simulink library "hEemethod"  (R2017b)
settings: Solver=VariableStepAuto  StartTime=0.0  StopTime=10.0  RelTol=1e-3
undefined symbols (not defined in the file or in its folder): Mag, r0_follower, v0_follower
libraries: hEemethod x13, vrlib x4, sharedutil x1, simulink x1
settings Model: Creator=mtwal  LastModifiedBy=mtwal
settings CodeAppCC: StateflowObjectComments=on

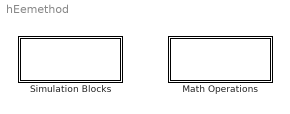
== system hEemethod ==
  Math Operations : Subsystem
  Simulation Blocks : Subsystem

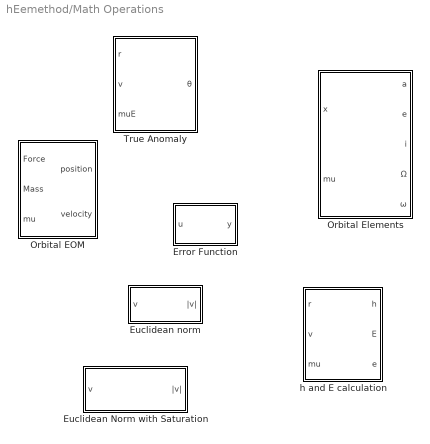
== system hEemethod/Math Operations ==
  Error Function : Subsystem  mask(Error Function){}
      mask help: Computes the error function of input signal u.
  Euclidean Norm with Saturation : Subsystem  mask(Euclidean Norm with Saturation){}
      mask help: Euclidean norm with minimum value of 1e-10 to avoid noise amplification at small values and maximum value of 1e20 to avoid infinity errors
  Euclidean norm : Subsystem  mask(Euclidean Norm){}
      mask help: Gives the Euclidean norm of a vector input
  Orbital EOM : Subsystem  mask(Orbit EOM){}
      mask help: Computes orbital EOM
  Orbital Elements : Subsystem  mask(Orbital Elements){}
      mask help: Calculates orbital elements from state vector x and gravitational constant mu
  True Anomaly : Subsystem  mask(True Anomaly){}
      mask help: Calculates true anomaly for given position, velocity, and planetary body
  h and E calculation : Subsystem  mask(hEe Calculation){}
      mask help: Calculate angular momentum (h), orbital energy (E), and eccentricity (e) for given postion, velocity, and gravitational constant

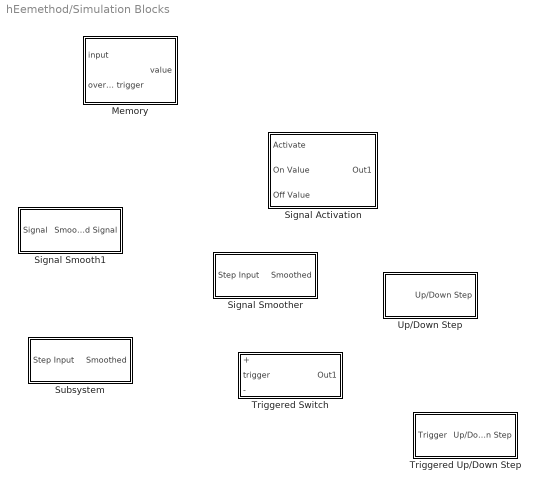
== system hEemethod/Simulation Blocks ==
  Memory : Subsystem  mask(Memory){}
      mask help: Holds value of input signal when a the value of overwrite trigger signal becomes greater than 0
  Signal Activation : Subsystem  mask(Signal Activation){RampTime=1}
      mask prompts: RampTime "Time for signal to ramp from 0 to 1"
      mask help: Outputs a signal that smoothly ramps from the off value to the on value when the activation input becomes greater than zero, and then smoothly ramps from the on value to the off value when the activation input becomes less than zero.
  Signal Smooth1 : Subsystem
  Signal Smoother : Subsystem  mask(Signal Smoother){Mag=0}
      mask prompts: Mag "Magnitude of Output Signal"
      mask help: Smooth a step function using an Error Function as a smooth approximation
  Subsystem : Subsystem
  Triggered Switch : Subsystem  mask(Triggered Switch){}
      mask help: Switches between + and - signal upon a triggering event
  Triggered Up/Down Step : Subsystem  mask(Triggered Up/Down Step){}
      mask help: Step up on rising trigger event and step down on falling trigger event
  Up/Down Step : Subsystem  mask(Up/Down Step){Mag1=0, tstep1=0, Mag2=0, tstep2=0}
      mask prompts: Mag1 "Magnitude of Positive Step Function"; tstep1 "Step Time of Positive Step Function"; Mag2 "Magnitude of Negative Step Function"; tstep2 "Step Time of Negative Step Function"
      mask help: Outputs a positive then a negative step function with specified magnitudes and step times.
      mask DialogControl Mag1 Tooltip: Magnitude of Positive Step
      mask DialogControl tstep1 Tooltip: Time of Positive Step
      mask DialogControl Mag2 Tooltip: Magnitude of Negative Step
      mask DialogControl tstep2 Tooltip: Step Time of Negative Step

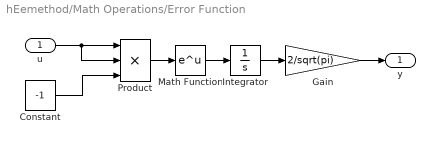
== system hEemethod/Math Operations/Error Function ==
  u : Inport
  Constant : Constant  Value=-1
  Gain : Gain  Gain=2/sqrt(pi)
  Integrator : Integrator
  Math Function : Math  SaturateOnIntegerOverflow=on
  Product : Product  Inputs=3
  y : Outport
  wires:
  u/1 -> Product/2, Product/1
  Constant/1 -> Product/3
  Product/1 -> Math Function/1
  Math Function/1 -> Integrator/1
  Integrator/1 -> Gain/1
  Gain/1 -> y/1

== system hEemethod/Math Operations/Euclidean Norm with Saturation ==
  v : Inport
  Dot Product : DotProduct  InputSameDT=on  OutDataTypeStr=Inherit: Inherit via internal rule
  Math Function : Math  Operator=sqrt  SaturateOnIntegerOverflow=on
  Saturation : Saturate  UpperLimit=1e20  LowerLimit=1e-10
  |v| : Outport
  wires:
  Saturation/1 -> |v|/1
  Math Function/1 -> Saturation/1
  v/1 -> Dot Product/1, Dot Product/2
  Dot Product/1 -> Math Function/1

== system hEemethod/Math Operations/Euclidean norm ==
  v : Inport
  Dot Product : DotProduct  InputSameDT=on  OutDataTypeStr=Inherit: Inherit via internal rule
  Math Function : Math  Operator=sqrt  SaturateOnIntegerOverflow=on
  |v| : Outport
  wires:
  v/1 -> Dot Product/1, Dot Product/2
  Dot Product/1 -> Math Function/1
  Math Function/1 -> |v|/1

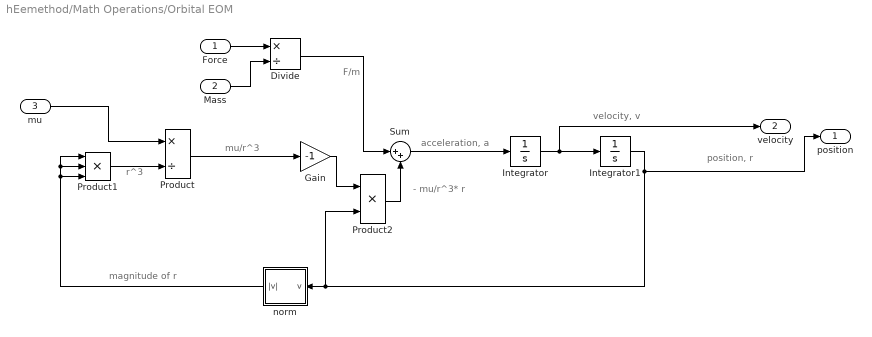
== system hEemethod/Math Operations/Orbital EOM ==
  note: F/m
  note: - mu/r^3* r
  note: mu/r^3
  note: r^3
  note: magnitude of r
  note: acceleration, a
  note: position, r
  note: velocity, v
  Force : Inport
  Mass : Inport  Port=2
  mu : Inport  Port=3
  Divide : Product  Inputs=*/
  Gain : Gain  Gain=-1  SaturateOnIntegerOverflow=on  OutDataTypeStr=Inherit: Same as input  ParamDataTypeStr=Inherit: Same as input
  Integrator : Integrator  InitialCondition=v0_follower  AbsoluteTolerance=1e-6
  Integrator1 : Integrator  InitialCondition=r0_follower  AbsoluteTolerance=1e-6
  Product : Product  Inputs=*/  SaturateOnIntegerOverflow=on  OutDataTypeStr=Inherit: Same as first input
  Product1 : Product  Inputs=***  SaturateOnIntegerOverflow=on  OutDataTypeStr=Inherit: Same as first input
  Product2 : Product  Inputs=**  SaturateOnIntegerOverflow=on  OutDataTypeStr=Inherit: Same as first input
  Sum : Sum  Inputs=|++
  norm : Subsystem
  position : Outport
  velocity : Outport  Port=2
  wires:
  mu/1 -> Product/1
  Product1/1 -> Product/2
  Integrator1/1 -> Product2/2, norm/1(v), position/1
  Product/1 -> Gain/1
  Integrator/1 -> Integrator1/1, velocity/1
  norm/1(|v|) -> Product1/1, Product1/2, Product1/3
  Gain/1 -> Product2/1
  Force/1 -> Divide/1
  Divide/1 -> Sum/1
  Product2/1 -> Sum/2
  Sum/1 -> Integrator/1
  Mass/1 -> Divide/2

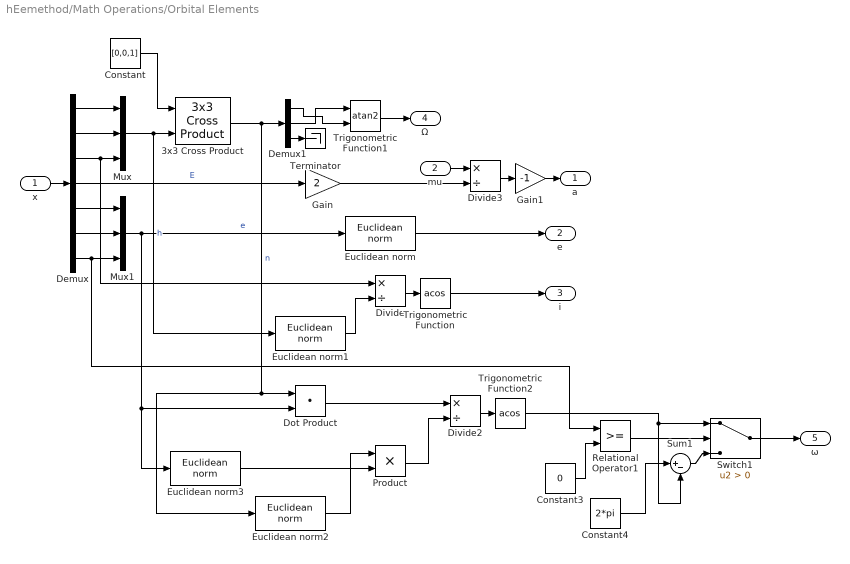
== system hEemethod/Math Operations/Orbital Elements ==
  x : Inport
  mu : Inport  Port=2
  3x3 Cross Product : sharedutil/3x3 Cross Product
      settings: SourceProductBaseCode=AE
  Constant : Constant  Value=[0,0,1]
  Constant3 : Constant  Value=0
  Constant4 : Constant  Value=2*pi
  Demux : Demux  Outputs=7
  Demux1 : Demux  Outputs=3
  Divide : Product  Inputs=*/
  Divide2 : Product  Inputs=*/
  Divide3 : Product  Inputs=*/
  Dot Product : DotProduct  InputSameDT=on  OutDataTypeStr=Inherit: Inherit via internal rule
  Euclidean norm{,1..3} (4 alike) : hEemethod/Math Operations/Euclidean norm
      settings: SourceProductName=HEe Method Library
  Gain : Gain  Gain=2
  Gain1 : Gain  Gain=-1
  Mux : Mux  Inputs=3
  Mux1 : Mux  Inputs=3
  Product : Product
  Relational Operator1 : RelationalOperator  OutDataTypeStr=boolean  RndMeth=Simplest
  Sum1 : Sum  Inputs=|+-
  Switch1 : Switch  Criteria=u2 > Threshold
  Terminator : Terminator
  Trigonometric Function : Trigonometry  Operator=acos
  Trigonometric Function1 : Trigonometry  Operator=atan2
  Trigonometric Function2 : Trigonometry  Operator=acos
  a : Outport
  e : Outport  Port=2
  i : Outport  Port=3
  Ω : Outport  Port=4
  ω : Outport  Port=5
  wires:
  Demux/1 -> Mux/1
  Demux/2 -> Mux/2
  Demux/3 -> Divide/1, Mux/3
  Demux/5 -> Mux1/1
  Demux/6 -> Mux1/2
  Demux/7 -> Relational Operator1/1, Mux1/3
  Demux/4 -> Gain/1  "E"
  Gain/1 -> Divide3/2
  Mux1/1 -> Euclidean norm/1, Euclidean norm3/1, Dot Product/2  "e"
  Euclidean norm/1 -> e/1
  Mux/1 -> Euclidean norm1/1, 3x3 Cross Product/2  "h"
  Constant/1 -> 3x3 Cross Product/1
  Divide/1 -> Trigonometric Function/1
  Euclidean norm1/1 -> Divide/2
  Trigonometric Function/1 -> i/1
  3x3 Cross Product/1 -> Demux1/1, Euclidean norm2/1, Dot Product/1  "n"
  Trigonometric Function1/1 -> Ω/1
  Euclidean norm3/1 -> Product/2
  Divide2/1 -> Trigonometric Function2/1
  Dot Product/1 -> Divide2/1
  Product/1 -> Divide2/2
  Sum1/1 -> Switch1/3
  Constant3/1 -> Relational Operator1/2
  Constant4/1 -> Sum1/1
  Relational Operator1/1 -> Switch1/2
  Switch1/1 -> ω/1
  Trigonometric Function2/1 -> Sum1/2, Switch1/1
  x/1 -> Demux/1
  mu/1 -> Divide3/1
  Gain1/1 -> a/1
  Divide3/1 -> Gain1/1
  Demux1/3 -> Terminator/1
  Demux1/2 -> Trigonometric Function1/1
  Demux1/1 -> Trigonometric Function1/2
  Euclidean norm2/1 -> Product/1

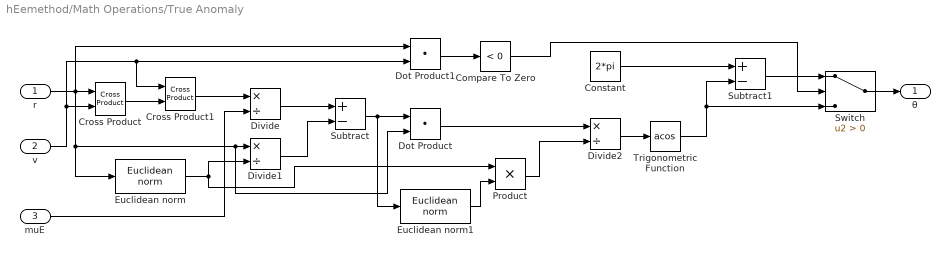
== system hEemethod/Math Operations/True Anomaly ==
  r : Inport
  v : Inport  Port=2
  muE : Inport  Port=3
  Compare To Zero : simulink/Logic and Bit Operations/Compare To Zero  relop=<  OutDataTypeStr=boolean
  Constant : Constant  Value=2*pi
  Cross Product : vrlib/Utilities/Cross Product
      settings: SourceProductBaseCode=VR
  Cross Product1 : vrlib/Utilities/Cross Product
      settings: SourceProductBaseCode=VR
  Divide : Product  Inputs=*/
  Divide1 : Product  Inputs=*/
  Divide2 : Product  Inputs=*/
  Dot Product : DotProduct  InputSameDT=on  OutDataTypeStr=Inherit: Inherit via internal rule
  Dot Product1 : DotProduct  InputSameDT=on  OutDataTypeStr=Inherit: Inherit via internal rule
  Euclidean norm : hEemethod/Math Operations/Euclidean norm
      settings: SourceProductName=HEe Method Library
  Euclidean norm1 : hEemethod/Math Operations/Euclidean norm
      settings: SourceProductName=HEe Method Library
  Product : Product
  Subtract : Sum  Inputs=+-
  Subtract1 : Sum  Inputs=+-
  Switch : Switch  Criteria=u2 > Threshold
  Trigonometric Function : Trigonometry  Operator=acos  OutputSignalType=real
  θ : Outport
  wires:
  r/1 -> Dot Product1/1, Dot Product/2, Divide1/1, Euclidean norm/1, Cross Product/1
  v/1 -> Cross Product/2, Cross Product1/1, Dot Product1/2
  Cross Product/1 -> Cross Product1/2
  Cross Product1/1 -> Divide/1
  muE/1 -> Divide/2
  Divide/1 -> Subtract/1
  Divide1/1 -> Subtract/2
  Euclidean norm/1 -> Product/1, Divide1/2
  Subtract/1 -> Euclidean norm1/1, Dot Product/1
  Dot Product/1 -> Divide2/1
  Product/1 -> Divide2/2
  Euclidean norm1/1 -> Product/2
  Dot Product1/1 -> Compare To Zero/1
  Constant/1 -> Subtract1/1
  Subtract1/1 -> Switch/1
  Compare To Zero/1 -> Switch/2
  Switch/1 -> θ/1
  Divide2/1 -> Trigonometric Function/1
  Trigonometric Function/1 -> Switch/3, Subtract1/2

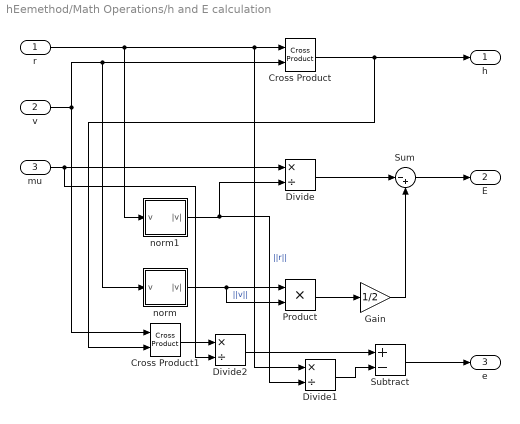
== system hEemethod/Math Operations/h and E calculation ==
  r : Inport
  v : Inport  Port=2
  mu : Inport  Port=3
  Cross Product : vrlib/Utilities/Cross Product
      settings: SourceProductBaseCode=VR
  Cross Product1 : vrlib/Utilities/Cross Product
      settings: SourceProductBaseCode=VR
  Divide : Product  Inputs=*/
  Divide1 : Product  Inputs=*/
  Divide2 : Product  Inputs=*/
  Gain : Gain  Gain=1/2
  Product : Product
  Subtract : Sum  Inputs=+-
  Sum : Sum  Inputs=|-+
  norm : Subsystem
  norm1 : Subsystem
  h : Outport
  E : Outport  Port=2
  e : Outport  Port=3
  wires:
  r/1 -> Divide1/1, Cross Product/1, norm1/1(v)
  v/1 -> Cross Product1/1, norm/1(v), Cross Product/2
  Cross Product/1 -> Cross Product1/2, h/1
  norm1/1(|v|) -> Divide1/2, Divide/2  "||r||"
  norm/1(|v|) -> Product/2, Product/1  "||v||"
  Product/1 -> Gain/1
  mu/1 -> Divide2/2, Divide/1
  Divide/1 -> Sum/1
  Gain/1 -> Sum/2
  Sum/1 -> E/1
  Divide1/1 -> Subtract/2
  Subtract/1 -> e/1
  Cross Product1/1 -> Divide2/1
  Divide2/1 -> Subtract/1

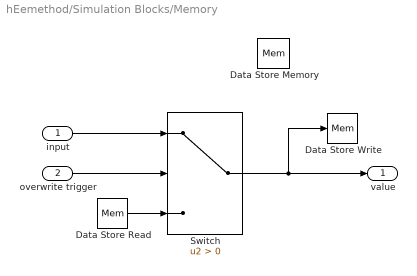
== system hEemethod/Simulation Blocks/Memory ==
  input : Inport
  overwrite trigger : Inport  Port=2
  Data Store Memory : DataStoreMemory  DataStoreName=Mem  ShowAdditionalParam=off
  Data Store Read : DataStoreRead  DataStoreName=Mem  SampleTime=[0,0]  DataStoreElements=Mem
  Data Store Write : DataStoreWrite  DataStoreName=Mem  SampleTime=[0,0]  DataStoreElements=Mem
  Switch : Switch  Criteria=u2 > Threshold
  value : Outport
  wires:
  Switch/1 -> Data Store Write/1, value/1
  input/1 -> Switch/1
  overwrite trigger/1 -> Switch/2
  Data Store Read/1 -> Switch/3

== system hEemethod/Simulation Blocks/Signal Activation ==
  Activate : Inport
  On Value : Inport  Port=2
  Off Value : Inport  Port=3
  Clock : Clock
  Memory : hEemethod/Simulation Blocks/Memory
      settings: SourceProductName=HEe Method Library
  Switch : Switch  Criteria=u2 > Threshold
  Out1 : Outport
  wires:
  Clock/1 -> ?
  Activate/1 -> Memory/2, Switch/2
  On Value/1 -> Switch/1
  Off Value/1 -> Switch/3
  Switch/1 -> Memory/1

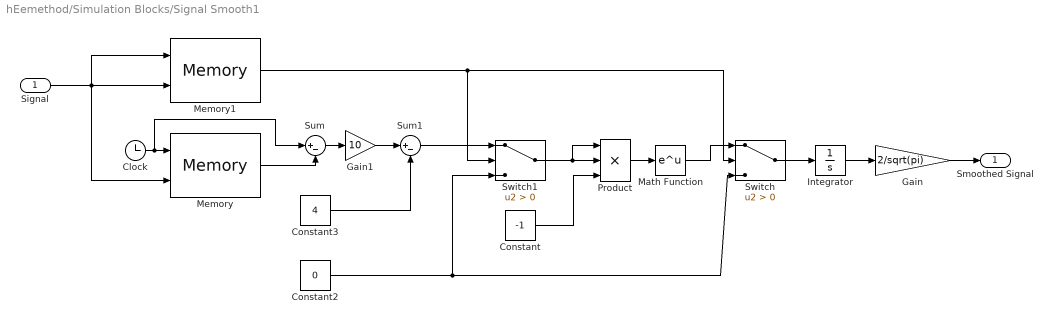
== system hEemethod/Simulation Blocks/Signal Smooth1 ==
  Signal : Inport
  Clock : Clock
  Constant : Constant  Value=-1
  Constant2 : Constant  Value=0
  Constant3 : Constant  Value=4
  Gain : Gain  Gain=2/sqrt(pi)
  Gain1 : Gain  Gain=10
  Integrator : Integrator
  Math Function : Math  SaturateOnIntegerOverflow=on
  Memory : hEemethod/Simulation Blocks/Memory
      settings: SourceProductName=HEe Method Library
  Memory1 : hEemethod/Simulation Blocks/Memory
      settings: SourceProductName=HEe Method Library
  Product : Product  Inputs=3
  Sum : Sum  Inputs=|+-
  Sum1 : Sum  Inputs=|+-
  Switch : Switch  Criteria=u2 > Threshold
  Switch1 : Switch  Criteria=u2 > Threshold
  Smoothed Signal : Outport
  wires:
  Memory/1 -> Sum/2
  Signal/1 -> Memory1/2, Memory1/1, Memory/2
  Clock/1 -> Sum/1, Memory/1
  Switch1/1 -> Product/1, Product/2
  Constant/1 -> Product/3
  Gain/1 -> Smoothed Signal/1
  Product/1 -> Math Function/1
  Integrator/1 -> Gain/1
  Switch/1 -> Integrator/1
  Math Function/1 -> Switch/1
  Memory1/1 -> Switch1/2, Switch/2
  Sum/1 -> Gain1/1
  Gain1/1 -> Sum1/1
  Sum1/1 -> Switch1/1
  Constant3/1 -> Sum1/2
  Constant2/1 -> Switch/3, Switch1/3

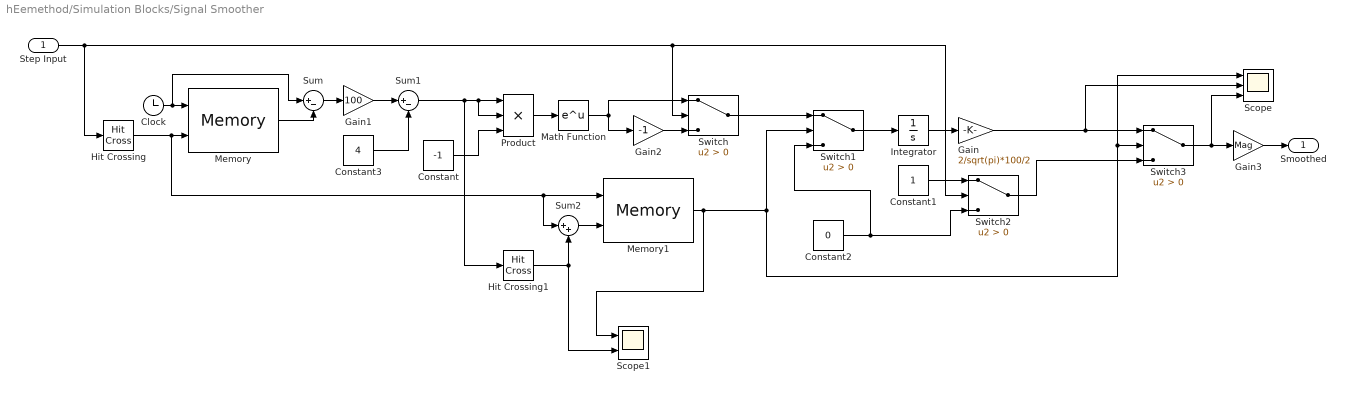
== system hEemethod/Simulation Blocks/Signal Smoother ==
  Step Input : Inport
  Clock : Clock
  Constant : Constant  Value=-1
  Constant1 : Constant
  Constant2 : Constant  Value=0
  Constant3 : Constant  Value=4
  Gain : Gain  Gain=2/sqrt(pi)*100/2
  Gain1 : Gain  Gain=100
  Gain2 : Gain  Gain=-1
  Gain3 : Gain  Gain=Mag
  Hit Crossing : HitCross  HitCrossingOffset=0.5
  Hit Crossing1 : HitCross  HitCrossingOffset=4  HitCrossingDirection=rising
  Integrator : Integrator
  Math Function : Math  SaturateOnIntegerOverflow=on
  Memory : hEemethod/Simulation Blocks/Memory
      settings: SourceProductName=HEe Method Library
  Memory1 : hEemethod/Simulation Blocks/Memory
      settings: SourceProductName=HEe Method Library
  Product : Product  Inputs=3
  Scope : Scope  NumInputPorts=3
  Scope1 : Scope  NumInputPorts=2
  Sum : Sum  Inputs=|+-
  Sum1 : Sum  Inputs=|+-
  Sum2 : Sum  Inputs=|++
  Switch{,1..3} (4 alike) : Switch  Criteria=u2 > Threshold
  Smoothed : Outport
  wires:
  Step Input/1 -> Hit Crossing/1, Switch/2, Switch2/2
  Product/1 -> Math Function/1
  Math Function/1 -> Gain2/1, Switch/1
  Integrator/1 -> Gain/1
  Clock/1 -> Sum/1, Memory/1
  Memory/1 -> Sum/2
  Constant/1 -> Product/3
  Constant3/1 -> Sum1/2
  Gain2/1 -> Switch/3
  Switch/1 -> Switch1/1
  Sum1/1 -> Hit Crossing1/1, Product/2, Product/1
  Switch3/1 -> Scope/3, Gain3/1
  Switch2/1 -> Switch3/3
  Constant1/1 -> Switch2/1
  Constant2/1 -> Switch1/3, Switch2/3
  Sum2/1 -> Memory1/2
  Hit Crossing/1 -> Sum2/1, Memory1/1, Memory/2
  Hit Crossing1/1 -> Scope1/2, Sum2/2
  Memory1/1 -> Scope1/1, Scope/1, Switch3/2, Switch1/2
  Switch1/1 -> Integrator/1
  Sum/1 -> Gain1/1
  Gain1/1 -> Sum1/1
  Gain/1 -> Scope/2, Switch3/1
  Gain3/1 -> Smoothed/1

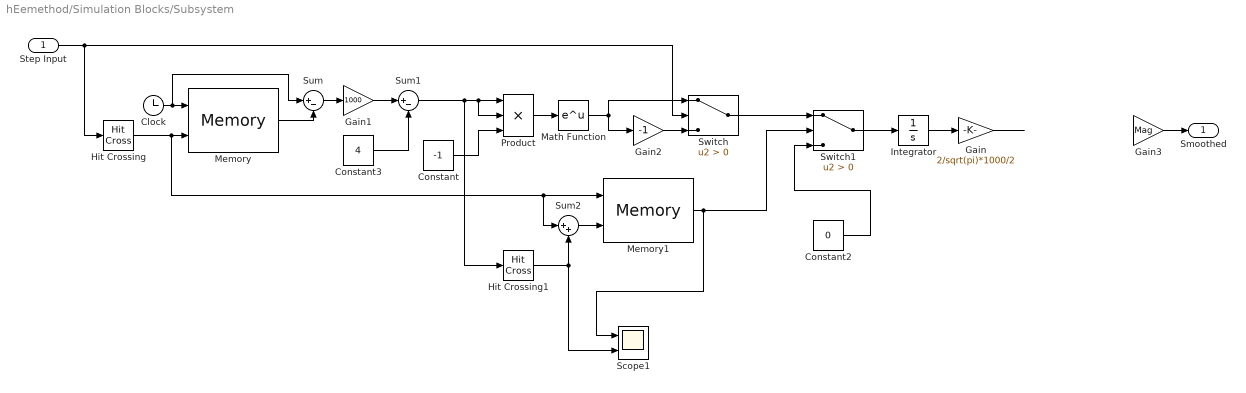
== system hEemethod/Simulation Blocks/Subsystem ==
  Step Input : Inport
  Clock : Clock
  Constant : Constant  Value=-1
  Constant2 : Constant  Value=0
  Constant3 : Constant  Value=4
  Gain : Gain  Gain=2/sqrt(pi)*1000/2
  Gain1 : Gain  Gain=1000
  Gain2 : Gain  Gain=-1
  Gain3 : Gain  Gain=Mag
  Hit Crossing : HitCross  HitCrossingOffset=0.5
  Hit Crossing1 : HitCross  HitCrossingOffset=4  HitCrossingDirection=rising
  Integrator : Integrator
  Math Function : Math  SaturateOnIntegerOverflow=on
  Memory : hEemethod/Simulation Blocks/Memory
      settings: SourceProductName=HEe Method Library
  Memory1 : hEemethod/Simulation Blocks/Memory
      settings: SourceProductName=HEe Method Library
  Product : Product  Inputs=3
  Scope1 : Scope  NumInputPorts=2
  Sum : Sum  Inputs=|+-
  Sum1 : Sum  Inputs=|+-
  Sum2 : Sum  Inputs=|++
  Switch : Switch  Criteria=u2 > Threshold
  Switch1 : Switch  Criteria=u2 > Threshold
  Smoothed : Outport
  wires:
  Gain3/1 -> Smoothed/1
  Switch/1 -> Switch1/1
  Constant2/1 -> Switch1/3
  Switch1/1 -> Integrator/1
  Step Input/1 -> Hit Crossing/1, Switch/2
  Hit Crossing/1 -> Sum2/1, Memory1/1, Memory/2
  Hit Crossing1/1 -> Scope1/2, Sum2/2
  Gain1/1 -> Sum1/1
  Memory1/1 -> Scope1/1, Switch1/2
  Sum1/1 -> Hit Crossing1/1, Product/2, Product/1
  Constant3/1 -> Sum1/2
  Sum/1 -> Gain1/1
  Gain/1 -> ?
  Gain2/1 -> Switch/3
  Product/1 -> Math Function/1
  Constant/1 -> Product/3
  Integrator/1 -> Gain/1
  Memory/1 -> Sum/2
  Clock/1 -> Sum/1, Memory/1
  Math Function/1 -> Gain2/1, Switch/1
  Sum2/1 -> Memory1/2

== system hEemethod/Simulation Blocks/Triggered Switch ==
  + : Inport
  trigger : Inport  Port=2
  - : Inport  Port=3
  Triggered Subsystem : Subsystem  TreatAsAtomicUnit=on
  Out1 : Outport
  wires:
  trigger/1 -> Triggered Subsystem/2(In3), Triggered Subsystem/Trigger
  +/1 -> Triggered Subsystem/1(In1)
  -/1 -> Triggered Subsystem/3(In2)
  Triggered Subsystem/1(Out1) -> Out1/1

== system hEemethod/Simulation Blocks/Triggered Up//Down Step ==
  Trigger : Inport
  Sum : Sum  Inputs=|++
  Triggered Subsystem : Subsystem  TreatAsAtomicUnit=on
  Triggered Subsystem1 : Subsystem  TreatAsAtomicUnit=on
  Up/Down Step : Outport
  wires:
  Sum/1 -> Up/Down Step/1
  Triggered Subsystem/1(Out1) -> Sum/1
  Triggered Subsystem1/1(Out1) -> Sum/2
  Trigger/1 -> Triggered Subsystem1/Trigger, Triggered Subsystem/Trigger

== system hEemethod/Simulation Blocks/Up//Down Step ==
  Step down : Step  Time=tstep2  After=-Mag2  SampleTime=0
  Step up : Step  Time=tstep1  After=Mag1  SampleTime=0
  Sum : Sum  Inputs=|++
  Up/Down Step : Outport
  wires:
  Step up/1 -> Sum/1
  Step down/1 -> Sum/2
  Sum/1 -> Up/Down Step/1

== system hEemethod/Math Operations/Orbital EOM/norm ==
  v : Inport
  Dot Product : DotProduct  InputSameDT=on  OutDataTypeStr=Inherit: Inherit via internal rule
  Math Function : Math  Operator=sqrt  SaturateOnIntegerOverflow=on
  Saturation : Saturate  UpperLimit=1e20  LowerLimit=1e-10
  |v| : Outport
  wires:
  v/1 -> Dot Product/1, Dot Product/2
  Dot Product/1 -> Math Function/1
  Math Function/1 -> Saturation/1
  Saturation/1 -> |v|/1

== system hEemethod/Math Operations/h and E calculation/norm ==
  v : Inport
  Dot Product : DotProduct  InputSameDT=on  OutDataTypeStr=Inherit: Inherit via internal rule
  Math Function : Math  Operator=sqrt  SaturateOnIntegerOverflow=on
  Saturation : Saturate  UpperLimit=1e20  LowerLimit=1e-10
  |v| : Outport
  wires:
  v/1 -> Dot Product/1, Dot Product/2
  Dot Product/1 -> Math Function/1
  Math Function/1 -> Saturation/1
  Saturation/1 -> |v|/1

== system hEemethod/Math Operations/h and E calculation/norm1 ==
  v : Inport
  Dot Product : DotProduct  InputSameDT=on  OutDataTypeStr=Inherit: Inherit via internal rule
  Math Function : Math  Operator=sqrt  SaturateOnIntegerOverflow=on
  Saturation : Saturate  UpperLimit=1e20  LowerLimit=1e-10
  |v| : Outport
  wires:
  v/1 -> Dot Product/1, Dot Product/2
  Dot Product/1 -> Math Function/1
  Math Function/1 -> Saturation/1
  Saturation/1 -> |v|/1

== system hEemethod/Simulation Blocks/Triggered Switch/Triggered Subsystem ==
  In1 : Inport
  In3 : Inport  Port=2
  In2 : Inport  Port=3
  Trigger : TriggerPort  TriggerType=either  VariantControl=Variant
  Switch : Switch  Criteria=u2 > Threshold
  Out1 : Outport
  wires:
  In1/1 -> Switch/1
  In2/1 -> Switch/3
  Switch/1 -> Out1/1
  In3/1 -> Switch/2

== system hEemethod/Simulation Blocks/Triggered Up//Down Step/Triggered Subsystem ==
  Trigger : TriggerPort  VariantControl=Variant
  Step up : Step  Time=0  SampleTime=0
  Out1 : Outport
  wires:
  Step up/1 -> Out1/1

== system hEemethod/Simulation Blocks/Triggered Up//Down Step/Triggered Subsystem1 ==
  Trigger : TriggerPort  TriggerType=falling  VariantControl=Variant
  Step : Step  Time=0  After=-1  SampleTime=0
  Out1 : Outport
  wires:
  Step/1 -> Out1/1
